simulink model "lab3"  (R2020b)
settings: Solver=FixedStepAuto  StartTime=0.0  StopTime=20.0  FixedStep=0.0001  RelTol=1e-3
InitFcn:
  | initialize
values from neighbouring files (symbols this model uses):
  A = [-0.12 0; 5 0]    [Assignment5.m]    (also in initialize.m)
  afDen = conv(fo,fo)    [initialize.m]
  B = [2.25; 0]    [Assignment5.m]    (also in initialize.m)
  C = [0 1]    [Assignment5.m]    (also in initialize.m = eye(2))
  D = 0    [Assignment5.m]    (also in initialize.m = [0;0])
  int_to_volt = volts/max_int10    (= 0.01953125)    [initialize.m]
  max_int10 = 2^(n_bits-1)    (= 512)    [initialize.m]
  ramp = 255    [initialize.m]
  rfq = 0.1    [initialize.m]
  volts = 10    [initialize.m]
libraries: simulink x3, simulink_extras x1
settings Model: Creator=claudio  LastModifiedBy=morri
settings SFSimCC: SimCustomHeaderCode="#include \"controllers.h\""  SimUserIncludeDirs=include
settings SFSimCC: SimUserSources=|
  | src/vel_float.c
  | src/pos_float.c
  | src/vel_fixed.c
  | src/pos_fixed.c

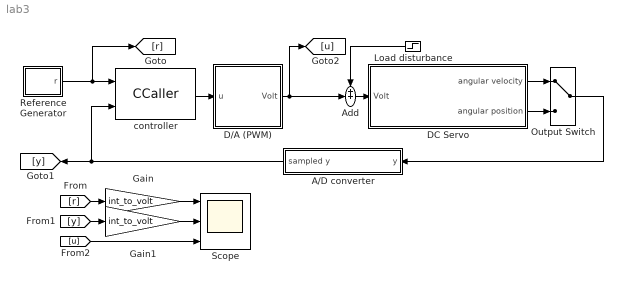
== system lab3 ==
  A/D converter : Subsystem
  Add : Sum  Inputs=++|
  D/A (PWM) : Subsystem
  "DC Servo " : Subsystem
  Gain : Gain  Gain=int_to_volt
  Gain1 : Gain  Gain=int_to_volt
  Load disturbance : Step  Time=12  After=1.5  SampleTime=0
  Output Switch : ManualSwitch
  Reference Generator : Subsystem
  Scope : Scope  NumInputPorts=3
  controller : CCaller  FunctionName=vel_fixed  PortSpecificationStruct="%)30     .    6 4   8    (     @         %    \"     ,    !     0         %  0 \"0    $    _    07)G3F%M90  4&]R=$YA;64 4V-O<&4     26YD97@     5'EP90      4VEZ90      27-';&]B86P   X    P    !@    @    $          4    (     0    ,    !         !   P!O=70 #@   #     &    \"     0         !0    @    !     P    $         $  # &]U=  .    .     8    (    !          %    \"     $    &     0         0    !@   $]U='!U=   #@   #@    &    \"     8         !0    @    !     0    $         \"0    @               X    X    !@    @    $          4    (     0    4    !         !     %    :6YT,38    .    ,     8    (    !          %    \"     $    !     0         0  $ ,0    X    P    !@    @    ) @        4    (     0    $    !          (  0      #@   #     &    \"     0         !0    @    !     0    $         $  ! '(    .    ,     8    (    !          %    \"     $    !     0         0  $ <@    X    X    !@    @    $          4    (     0    4    !         !     %    26YP=70    .    .     8    (    !@         %    \"     $    !     0         )    \"               #@   #@    &    \"     0         !0    @    !    !0    $         $     4   !I;G0Q-@    X    P    !@    @    $          4    (     0    $    !         !   0 Q    #@   #     &    \"     D\"        !0    @    !     0    $          @ !       .    ,     8    (    !          %    \"     $    !     0         0  $ >0    X    P    !@    @    $          4    (     0    $    !         !   0!Y    #@   #@    &    \"     0         !0    @    !    !0    $         $     4   !);G!U=     X    X    !@    @    &          4    (     0    $    !          D    (            \\#\\.    .     8    (    !          %    \"     $    %     0         0    !0   &EN=#$V    #@   #     &    \"     0         !0    @    !     0    $         $  ! #$    .    ,     8    (    \"0(        %    \"     $    !     0         \"  $"
  wires:
  Gain/1 -> Scope/1
  Gain1/1 -> Scope/2
  [u] -> Scope/3
  Reference Generator/1(r) -> [r], controller/1
  [r] -> Gain/1
  [y] -> Gain1/1
  "DC Servo "/1(angular velocity) -> Output Switch/1
  "DC Servo "/2(angular position) -> Output Switch/2
  controller/1 -> D/A (PWM)/1(u)
  Add/1 -> "DC Servo "/1(Volt)
  A/D converter/1(sampled y) -> controller/2, [y]
  Output Switch/1 -> A/D converter/1(y)
  D/A (PWM)/1(Volt) -> Add/2, [u]
  Load disturbance/1 -> Add/1

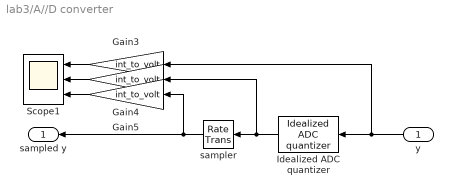
== system lab3/A//D converter ==
  y : Inport
  Gain3 : Gain  Gain=int_to_volt
  Gain4 : Gain  Gain=int_to_volt
  Gain5 : Gain  Gain=int_to_volt
  Idealized ADC quantizer : simulink_extras/Additional Discrete/Idealized ADC quantizer  NumberOfConverterBits=n_bits  Vmin=-512  Vmax=511  OutputDataType=int16  OutputNegativeValues=on
  Scope1 : Scope  NumInputPorts=3
  sampler : RateTransition  OutPortSampleTime=st
  sampled y : Outport
  wires:
  Gain4/1 -> Scope1/2
  Gain3/1 -> Scope1/1
  sampler/1 -> sampled y/1, Gain5/1
  Idealized ADC quantizer/1 -> Gain4/1, sampler/1
  Gain5/1 -> Scope1/3
  y/1 -> Gain3/1, Idealized ADC quantizer/1

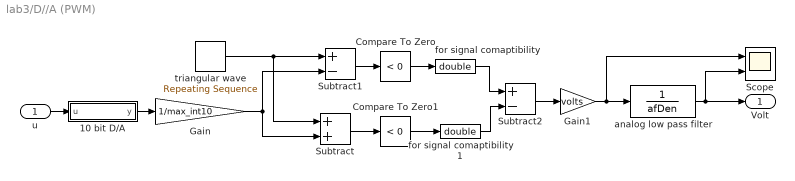
== system lab3/D//A (PWM) ==
  u : Inport
  10 bit D/A : MATLAB Function  TreatAsAtomicUnit=on
  Compare To Zero : simulink/Logic and Bit Operations/Compare To Zero  relop=<  OutDataTypeStr=boolean
  Compare To Zero1 : simulink/Logic and Bit Operations/Compare To Zero  relop=<  OutDataTypeStr=boolean
  Gain : Gain  Gain=1/max_int10
  Gain1 : Gain  Gain=volts
  Scope : Scope  NumInputPorts=2
  Subtract : Sum
  Subtract1 : Sum  Inputs=+-
  Subtract2 : Sum  Inputs=+-
  analog low pass filter : TransferFcn  Numerator=1  Denominator=afDen
  for signal comaptibility : DataTypeConversion  OutMin=[-512]  OutMax=[511]  OutDataTypeStr=double
  for signal comaptibility1 : DataTypeConversion  OutMin=[-512]  OutMax=[511]  OutDataTypeStr=double
  triangular wave : simulink/Sources/Repeating Sequence  rep_seq_t=[0 0.01]  rep_seq_y=[0 1]
  Volt : Outport
  wires:
  u/1 -> 10 bit D/A/1(u)
  10 bit D/A/1(y) -> Gain/1
  Subtract1/1 -> Compare To Zero/1
  Subtract2/1 -> Gain1/1
  Compare To Zero1/1 -> for signal comaptibility1/1
  Compare To Zero/1 -> for signal comaptibility/1
  for signal comaptibility/1 -> Subtract2/1
  analog low pass filter/1 -> Volt/1, Scope/2
  Subtract/1 -> Compare To Zero1/1
  for signal comaptibility1/1 -> Subtract2/2
  triangular wave/1 -> Subtract/1, Subtract1/1
  Gain/1 -> Subtract1/2, Subtract/2
  Gain1/1 -> analog low pass filter/1, Scope/1

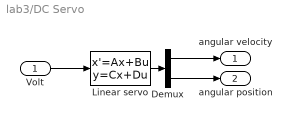
== system lab3/DC Servo  ==
  Volt : Inport
  Demux : Demux  Outputs=2
  Linear servo : StateSpace  A=A  B=B*max_int10/10  C=C  D=D  InitialCondition=[0,0]
  angular velocity : Outport
  angular position : Outport  Port=2
  wires:
  Demux/1 -> angular velocity/1
  Demux/2 -> angular position/1
  Linear servo/1 -> Demux/1
  Volt/1 -> Linear servo/1

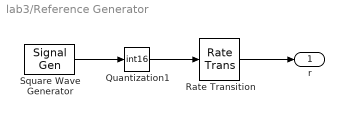
== system lab3/Reference Generator ==
  Quantization1 : DataTypeConversion  OutMin=[-512]  OutMax=[511]  OutDataTypeStr=int16
  Rate Transition : RateTransition  OutPortSampleTime=st
  Square Wave Generator : SignalGenerator  WaveForm=square  Amplitude=ramp  Frequency=rfq
  r : Outport
  wires:
  Square Wave Generator/1 -> Quantization1/1
  Rate Transition/1 -> r/1
  Quantization1/1 -> Rate Transition/1

== matlab function lab3/D//A (PWM)/10 bit D//A ==
  data: u input; y output
% this function emiulates the fact of having
% a 10 bits D/A converter that can cause sign 
% inversion in case of overflow 

function y = fcn(u)

if u>511
    y = -512+(u-511);
    return
elseif u<-512
    y = -(u+512);
    return
end

y=u;

end
